simulink model "half_wave_rectifier"  (R2020a)
settings: Solver=VariableStepAuto  StartTime=0.0  StopTime=0.1  RelTol=1e-3
settings Model: Creator=Ganesh  LastModifiedBy=Ganesh

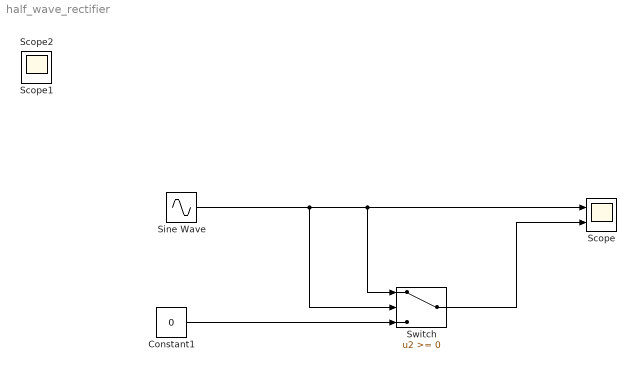
== system half_wave_rectifier ==
  Constant1 : Constant  Value=0  SampleTime=1e-6
  Scope : Scope  NumInputPorts=2
  Sine Wave : Sin  Frequency=50*pi*2  SampleTime=0
  Switch : Switch
  Scope1 : Scope
  Scope2 : Scope
  wires:
  Sine Wave/1 -> Switch/1, Scope/1, Switch/2
  Constant1/1 -> Switch/3
  Switch/1 -> Scope/2
